simulink model "sampleModel312"  (R2021b)
settings: Solver=VariableStepAuto  StartTime=0.0  StopTime=10.0  RelTol=1e-3
libraries: simulink x3, slpidlib x1
settings Model: Creator=user  LastModifiedBy=user

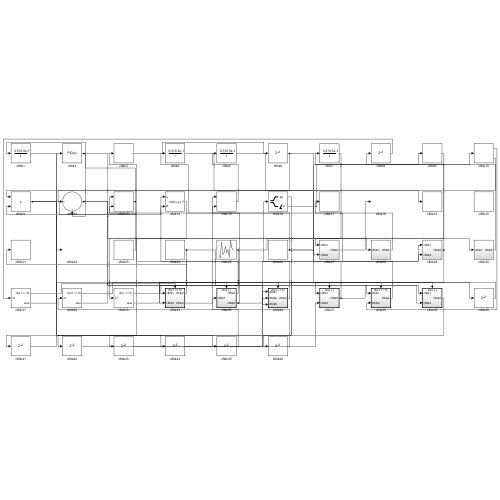
[thumbnail: Simulink's stored preview of the top-level diagram]
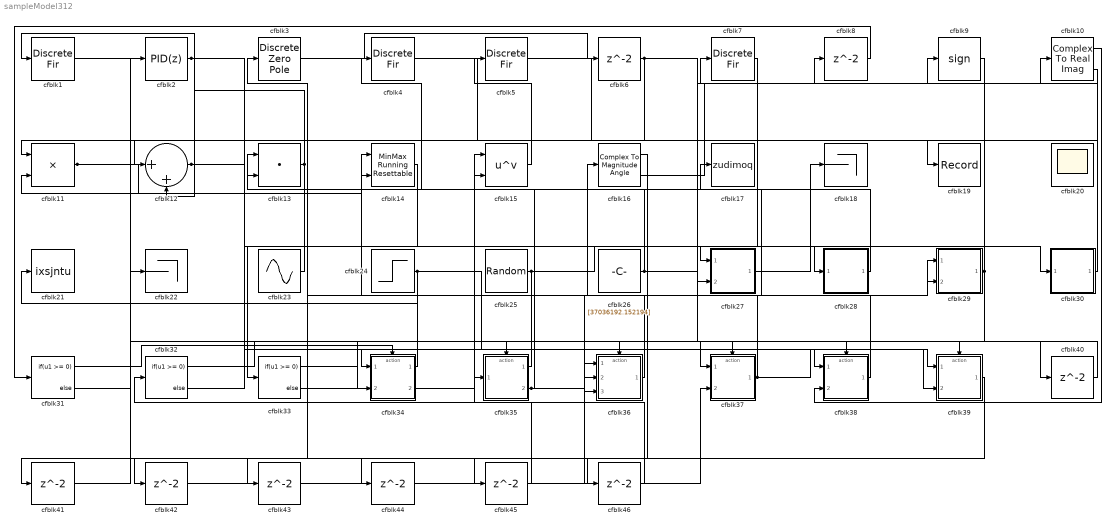
== system sampleModel312 ==
  cfblk{1,4..5,7} (4 alike) : DiscreteFir  SampleTime=1
  cfblk10 : ComplexToRealImag
  cfblk11 : Product  Inputs=**
  cfblk12 : Sum  Inputs=|++
  cfblk13 : DotProduct  InputSameDT=on  OutDataTypeStr=Inherit: Inherit via internal rule
  cfblk14 : simulink/Math Operations/MinMax Running Resettable  Function=min  vinit=0.0
  cfblk15 : Math  Operator=pow  SaturateOnIntegerOverflow=on
  cfblk16 : ComplexToMagnitudeAngle
  cfblk17 : ToWorkspace  VariableName=zudimoq  SaveFormat=Timeseries  SampleTime=-1
  cfblk18 : Terminator
  cfblk19 : Record  FileSettingsInternal="{\"entries\":[{\"content\":{\"excelSettings\":{\"content\":{},\"type\":\"Streamout.ExcelSettings\"}},\"type\":\"Streamout.FileSettingStorage\",\"uuid\":\"9ac1a609-0274-40f3-95ac-3884fedccbc3\"}],\"packageUris\":[\"http://schema.mathworks.com/mf0/streamout_blocks/R2020a\"],\"version\":\"1.0\"}"  SignalsInternal="{\"entries\":[{\"content\":{\"signals\":[{\"content\":{\"blockPath\":[\"sampleModel312/cfblk19\"],\"channel\":[],\"dimensions\":[1],\"domain\":\"sampleModel312/cfblk19\",\"lineColor\":\"#ff6929\",\"plots\":[1],\"port\":1,\"sid\":[\"\"],\"signalID\":13197,\"signalName\":\"cfblk5\"},\"type\":\"RecordBlkView.Signal\",\"uuid\":\"3e87320b-8d94-4d69-95d8-2f6ff7c5ef6c\"}]},\"type\":\"RecordBlkView.InputSignals\",\"uuid\":\"46d423cf-9168-483a-8ef6-76ee166d89ca\"}],\"packageUris\":[\"http://schema.mathworks.com/mf0/streamout_blocks/R2020a\"],\"version\":\"1.0\"}"  VisualizationBindings="{\"sparklinesplugin\":{\"info\":[{\"bindingParametersList\":[],\"subplotID\":1}]}}"
  cfblk2 : slpidlib/PID Controller  Controller=PID  Form=Parallel  TimeDomain=Discrete-time  UseExternalTs=off  SampleTime=1  IntegratorMethod=Forward Euler  FilterMethod=Forward Euler  ControllerParametersSource=internal  P=1  I=1  D=0  UseFilter=on  N=100  TunerSelectOption=Transfer Function Based (PID Tuner App)  InitialConditionSource=internal  InitialConditionForIntegrator=0  InitialConditionForFilter=0  DifferentiatorICPrevScaledInput=0  ExternalReset=none  TrackingMode=off  Kt=1  LimitOutput=off  SatLimitsSource=internal  UpperSaturationLimit=inf  LowerSaturationLimit=-inf  LinearizeAsGain=off  AntiWindupMode=none  Kb=1  POutMin=[]  POutMax=[]  IOutMin=[]  IOutMax=[]  DOutMin=[]  DOutMax=[]  NOutMin=[]  NOutMax=[]  SumOutMin=[]  SumOutMax=[]  SaturationOutMin=[]  SaturationOutMax=[]  PParamMin=[]  PParamMax=[]  IParamMin=[]  IParamMax=[]  DParamMin=[]  DParamMax=[]  NParamMin=[]  NParamMax=[]  KbParamMin=[]  KbParamMax=[]  KtParamMin=[]  KtParamMax=[]  KbOutMin=[]  KbOutMax=[]  KtOutMin=[]  KtOutMax=[]  IntegratorOutMin=[]  IntegratorOutMax=[]  FilterOutMin=[]  FilterOutMax=[]  SumI1OutMin=[]  SumI1OutMax=[]  SumI2OutMin=[]  SumI2OutMax=[]  SumI3OutMin=[]  SumI3OutMax=[]  SumI4OutMin=[]  SumI4OutMax=[]  SumDOutMin=[]  SumDOutMax=[]  DifferentiatorOutMin=[]  DifferentiatorOutMax=[]  FilterDiffOutCoefMin=[]  FilterDiffOutCoefMax=[]  ReciprocalOutMin=[]  ReciprocalOutMax=[]  SumDenOutMin=[]  SumDenOutMax=[]  SumNumOutMin=[]  SumNumOutMax=[]  DivideOutMin=[]  DivideOutMax=[]  UdiffTsProdOutMin=[]  UdiffTsProdOutMax=[]  NTsProdOutMin=[]  NTsProdOutMax=[]  UintegralTsProdOutMin=[]  UintegralTsProdOutMax=[]  UngainTsProdOutMin=[]  UngainTsProdOutMax=[]  IntegratorContinuousStateAttributes=''  IntegratorStateMustResolveToSignalObject=off  IntegratorRTWStateStorageClass=Auto  FilterContinuousStateAttributes=''  FilterStateMustResolveToSignalObject=off  FilterRTWStateStorageClass=Auto  ParallelPVariant=InternalParameters  IdealPVariant=Disabled  IVariant=InternalParameters  DVariant=InternalParameters  IntegratorVariant=Discrete  SatVariant=Disabled  AWVariant=Passthrough  PCopyVariant=Disabled  TRVariant=Disabled  FdbkBlocksVariant=Forward  IdealPFdbkVariant=Disabled  SatFdbkVariant=Disabled  DerivativeFilterVariant=ForwardEulerFilter  NVariant=InternalParameters  NCopyVariant=Disabled  FilterICVariant=InternalICsFilter  IntegratorICVariant=InternalICs  ExternalResetVariant=Disabled  TRSumVariant=Passthrough  SumFdbkVariant=Disabled  SumVariant=Sum_PID  TsampFilterVariant=InternalTs  TsampNgainVariant=Passthrough  TsampIntegralVariant=Passthrough  ExternalSaturationOutDataTypeStr=Inherit: Same as second input
  cfblk20 : Scope
      settings: Floating=on
  cfblk21 : ToWorkspace  VariableName=ixsjntu  SaveFormat=Timeseries  SampleTime=-1
  cfblk22 : Terminator
  cfblk23 : Sin  Amplitude=[746673708.938308]  Bias=[-649272381.164565]  SampleTime=0
  cfblk24 : Step  Time=[35.000000]  Before=[474305.216489]  After=[-134711307.131538]  SampleTime=0
  cfblk25 : UniformRandomNumber  Minimum=[-6027552277.649668]  Maximum=[2086321643.267048]  Seed=[30243039.000000]  SampleTime=0.1
  cfblk26 : Constant  Value=[37036192.152194]  SampleTime=1
  cfblk27 : Subsystem
  cfblk28 : Subsystem
  cfblk29 : Subsystem
  cfblk3 : DiscreteZeroPole  Poles=[0 0.5]  Gain=1
  cfblk30 : Subsystem
  cfblk31 : If  IfExpression=u1 >= 0  SampleTime=1
  cfblk32 : If  IfExpression=u1 >= 0  SampleTime=1
  cfblk33 : If  IfExpression=u1 >= 0  SampleTime=1
  cfblk34 : Subsystem  TreatAsAtomicUnit=on
  cfblk35 : Subsystem  TreatAsAtomicUnit=on
  cfblk36 : Subsystem  TreatAsAtomicUnit=on
  cfblk37 : Subsystem  TreatAsAtomicUnit=on
  cfblk38 : Subsystem  TreatAsAtomicUnit=on
  cfblk39 : Subsystem  TreatAsAtomicUnit=on
  cfblk{6,8,40..46} (9 alike) : Delay  SampleTime=1
  cfblk9 : Signum
  wires:
  cfblk25/1 -> cfblk28/1(cfblk1), cfblk34/1(cfblk1)
  cfblk30/1(cfblk2) -> cfblk8/1
  cfblk28/1(cfblk2) -> cfblk15/1
  cfblk34/1(cfblk2) -> cfblk21/1
  cfblk5/1 -> cfblk19/1
  cfblk34/2(cfblk4) -> cfblk15/2
  cfblk6/1 -> cfblk12/1, cfblk40/1
  cfblk24/1 -> cfblk38/1(cfblk1), cfblk34/2(cfblk3)
  cfblk35/1(cfblk2) -> cfblk14/1
  cfblk10/1 -> cfblk38/2(cfblk4)
  cfblk23/1 -> cfblk13/1
  cfblk37/1(cfblk2) -> cfblk39/1(cfblk1), cfblk16/1
  cfblk36/1(cfblk2) -> cfblk3/1
  cfblk9/1 -> cfblk27/1(cfblk1)
  cfblk27/1(cfblk2) -> cfblk18/1
  cfblk4/1 -> cfblk27/2(cfblk3)
  cfblk13/1 -> cfblk1/1, cfblk11/2
  cfblk15/1 -> cfblk5/1
  cfblk16/2 -> cfblk9/1
  cfblk11/1 -> cfblk14/2, cfblk44/1, cfblk45/1
  cfblk35/2(cfblk5) -> cfblk13/2, cfblk29/1(cfblk1)
  cfblk12/1 -> cfblk39/2(cfblk3), cfblk30/1(cfblk1)
  cfblk10/2 -> cfblk11/1
  cfblk29/1(cfblk2) -> cfblk7/1, cfblk46/1
  cfblk7/1 -> cfblk33/1
  cfblk38/1(cfblk2) -> cfblk17/1
  cfblk2/1 -> cfblk36/3(cfblk5), cfblk12/2
  cfblk8/1 -> cfblk31/1
  cfblk3/1 -> cfblk6/1
  cfblk26/1 -> cfblk4/1, cfblk10/1, cfblk29/2(cfblk4)
  cfblk1/1 -> cfblk22/1
  cfblk31/1 -> cfblk34/Action
  cfblk31/2 -> cfblk35/Action
  cfblk32/1 -> cfblk36/Action
  cfblk32/2 -> cfblk37/Action
  cfblk33/1 -> cfblk38/Action
  cfblk33/2 -> cfblk39/Action
  cfblk40/1 -> cfblk37/1(cfblk1)
  cfblk39/1(cfblk2) -> cfblk41/1
  cfblk41/1 -> cfblk2/1
  cfblk16/1 -> cfblk42/1
  cfblk42/1 -> cfblk36/1(cfblk1)
  cfblk14/1 -> cfblk43/1
  cfblk43/1 -> cfblk36/2(cfblk4)
  cfblk44/1 -> cfblk37/2(cfblk5)
  cfblk45/1 -> cfblk32/1
  cfblk46/1 -> cfblk35/1(cfblk1)

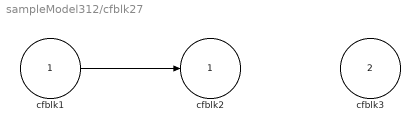
== system sampleModel312/cfblk27 ==
  cfblk1 : Inport
  cfblk3 : Inport  Port=2
  cfblk2 : Outport
  wires:
  cfblk1/1 -> cfblk2/1

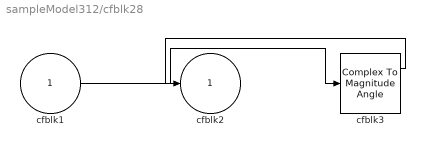
== system sampleModel312/cfblk28 ==
  cfblk1 : Inport
  cfblk3 : ComplexToMagnitudeAngle
  cfblk2 : Outport
  wires:
  cfblk1/1 -> cfblk3/1
  cfblk3/1 -> cfblk2/1

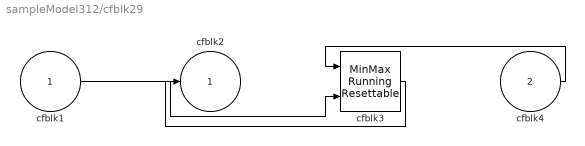
== system sampleModel312/cfblk29 ==
  cfblk1 : Inport
  cfblk4 : Inport  Port=2
  cfblk3 : simulink/Math Operations/MinMax Running Resettable  Function=min  vinit=0.0
  cfblk2 : Outport
  wires:
  cfblk4/1 -> cfblk3/1
  cfblk1/1 -> cfblk3/2
  cfblk3/1 -> cfblk2/1

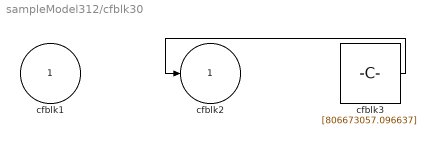
== system sampleModel312/cfblk30 ==
  cfblk1 : Inport
  cfblk3 : Constant  Value=[806673057.096637]  SampleTime=1
  cfblk2 : Outport
  wires:
  cfblk3/1 -> cfblk2/1

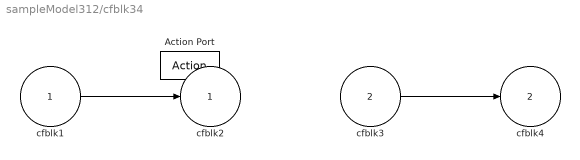
== system sampleModel312/cfblk34 ==
  cfblk1 : Inport
  cfblk3 : Inport  Port=2
  Action Port : ActionPort  ActionPortLabel=if(u1 >= 0)
  cfblk2 : Outport
  cfblk4 : Outport  Port=2
  wires:
  cfblk3/1 -> cfblk4/1
  cfblk1/1 -> cfblk2/1

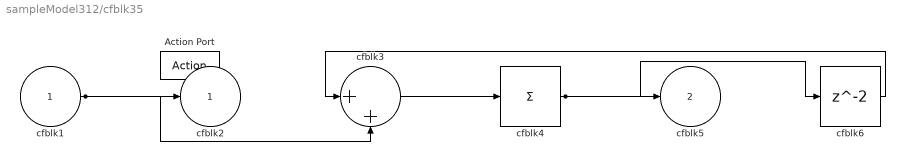
== system sampleModel312/cfblk35 ==
  cfblk1 : Inport
  Action Port : ActionPort  ActionPortLabel=else
  cfblk3 : Sum  Inputs=|++
  cfblk4 : Sum  Inputs=+
  cfblk6 : Delay
  cfblk2 : Outport
  cfblk5 : Outport  Port=2
  wires:
  cfblk3/1 -> cfblk4/1
  cfblk1/1 -> cfblk2/1, cfblk3/2
  cfblk4/1 -> cfblk5/1, cfblk6/1
  cfblk6/1 -> cfblk3/1

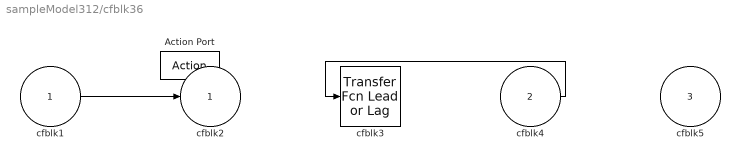
== system sampleModel312/cfblk36 ==
  cfblk1 : Inport
  cfblk4 : Inport  Port=2
  cfblk5 : Inport  Port=3
  Action Port : ActionPort  ActionPortLabel=if(u1 >= 0)
  cfblk3 : simulink/Discrete/Transfer Fcn Lead or Lag  PoleZ=0.95  ZeroZ=0.75  ICPrevOutput=0.0  ICPrevInput=0.0  DoSatur=off
      settings: SourceProductBaseCode=SL
  cfblk2 : Outport
  wires:
  cfblk1/1 -> cfblk2/1
  cfblk4/1 -> cfblk3/1

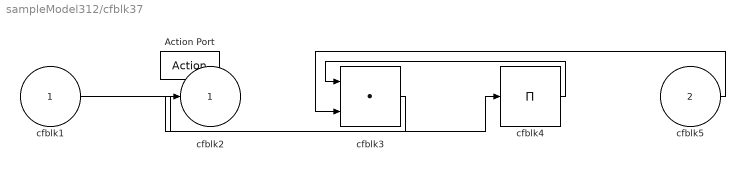
== system sampleModel312/cfblk37 ==
  cfblk1 : Inport
  cfblk5 : Inport  Port=2
  Action Port : ActionPort  ActionPortLabel=else
  cfblk3 : DotProduct  InputSameDT=on  OutDataTypeStr=Inherit: Inherit via internal rule
  cfblk4 : Product  Inputs=*
  cfblk2 : Outport
  wires:
  cfblk1/1 -> cfblk4/1
  cfblk4/1 -> cfblk3/1
  cfblk3/1 -> cfblk2/1
  cfblk5/1 -> cfblk3/2

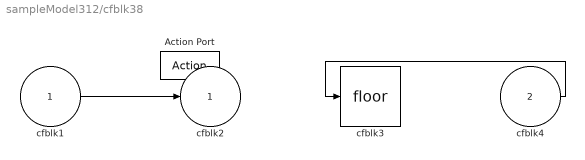
== system sampleModel312/cfblk38 ==
  cfblk1 : Inport
  cfblk4 : Inport  Port=2
  Action Port : ActionPort  ActionPortLabel=if(u1 >= 0)
  cfblk3 : Rounding
  cfblk2 : Outport
  wires:
  cfblk4/1 -> cfblk3/1
  cfblk1/1 -> cfblk2/1

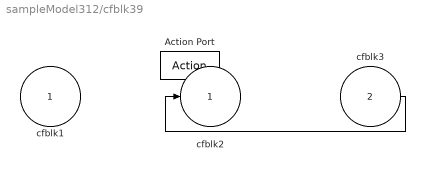
== system sampleModel312/cfblk39 ==
  cfblk1 : Inport
  cfblk3 : Inport  Port=2
  Action Port : ActionPort  ActionPortLabel=else
  cfblk2 : Outport
  wires:
  cfblk3/1 -> cfblk2/1
